simulink model "single_pendulum_R2018b"  (R2018b)
settings: Solver=ode1  StartTime=0.0  StopTime=60  FixedStep=0.01  MaxStep=0.1  RelTol=1e-3
settings Model: EnablePacing=on  Creator=mojo  LastModifiedBy=mojo
settings DataIOCC: ReturnWorkspaceOutputs=on

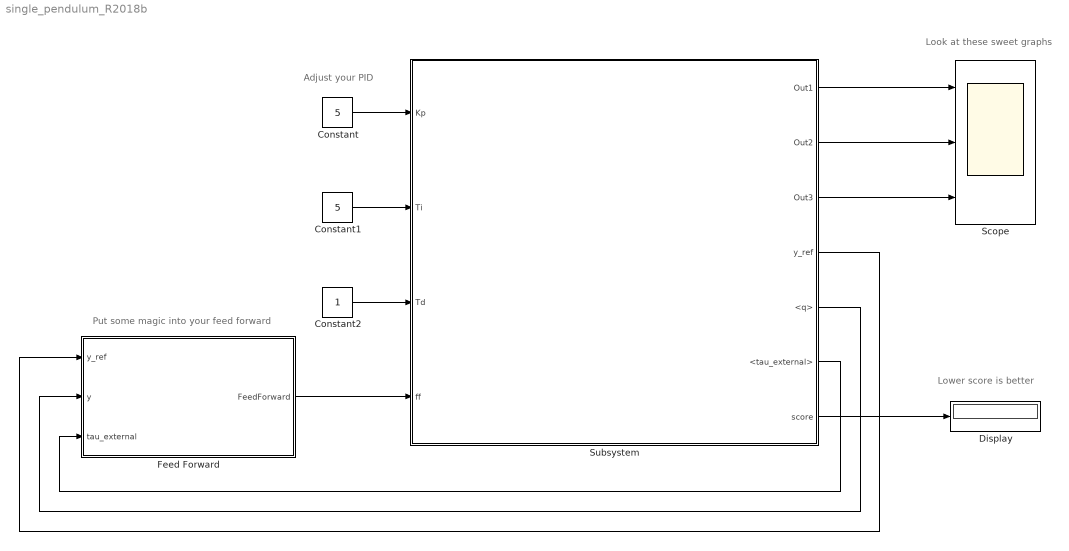
== system single_pendulum_R2018b ==
  note: Look at these sweet graphs
  note: Adjust your PID
  note: Put some magic into your feed forward
  note: Lower score is better
  Constant : Constant  Value=5
  Constant1 : Constant  Value=5
  Constant2 : Constant
  Display : Display
  Feed Forward : MATLAB Function  TreatAsAtomicUnit=on
  Scope : Scope  NumInputPorts=3
  Subsystem : Subsystem
  wires:
  Constant/1 -> Subsystem/1(Kp)
  Constant1/1 -> Subsystem/2(Ti)
  Constant2/1 -> Subsystem/3(Td)
  Feed Forward/1(FeedForward) -> Subsystem/4(ff)
  Subsystem/1(Out1) -> Scope/1
  Subsystem/2(Out2) -> Scope/2
  Subsystem/3(Out3) -> Scope/3
  Subsystem/4(y_ref) -> Feed Forward/1(y_ref)
  Subsystem/5(<q>) -> Feed Forward/2(y)
  Subsystem/6(<tau_external>) -> Feed Forward/3(tau_external)
  Subsystem/7(score) -> Display/1

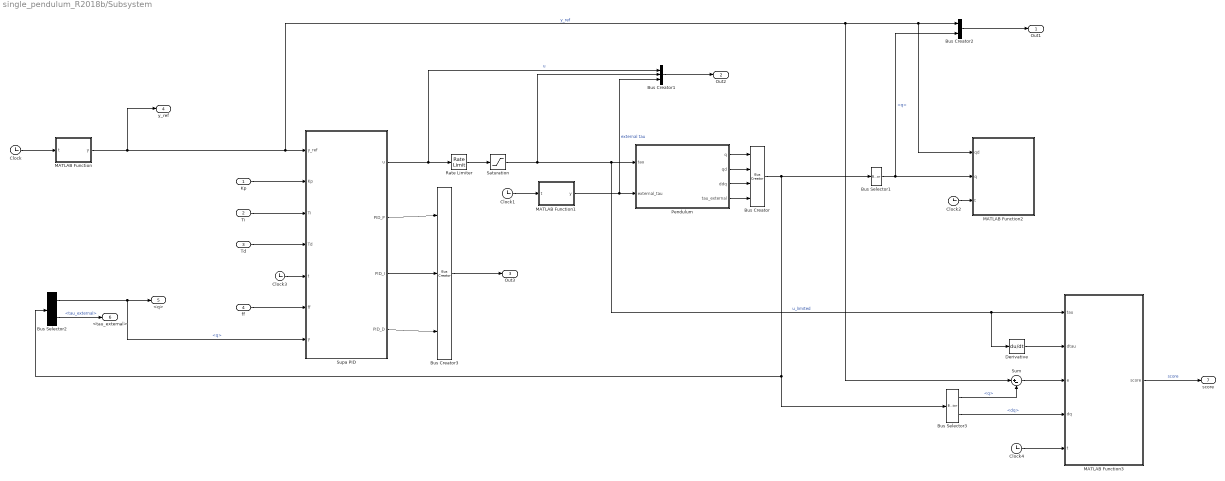
== system single_pendulum_R2018b/Subsystem ==
  Kp : Inport
  Ti : Inport  Port=2
  Td : Inport  Port=3
  ff : Inport  Port=4
  Bus Creator : BusCreator  Inputs=4
  Bus Creator1 : BusCreator  Inputs=3
  Bus Creator2 : BusCreator  Inputs=2
  Bus Creator3 : BusCreator  Inputs=3
  Bus Selector1 : BusSelector  OutputSignals=q
  Bus Selector2 : BusSelector  OutputSignals=q,tau_external
  Bus Selector3 : BusSelector  OutputSignals=q,dq
  Clock{,1..4} (5 alike) : Clock
  Derivative : Derivative
  MATLAB Function : MATLAB Function  TreatAsAtomicUnit=on
  MATLAB Function1 : MATLAB Function  TreatAsAtomicUnit=on
  MATLAB Function2 : MATLAB Function  TreatAsAtomicUnit=on
  MATLAB Function3 : MATLAB Function  TreatAsAtomicUnit=on
  Pendulum : Subsystem  mask{I=1, q_0=pi/2, Mass=1, Length=1, g=9.81, B=1}
      mask prompts: I "Inertia [kg*m]"; q_0 "Initial position [rad]"; Mass "Mass [kg]"; Length "Length [m]"; g "g [m/s^2]"; B "Friction [kg/s]"
  Rate Limiter : RateLimiter  RisingSlewLimit=20  FallingSlewLimit=-20  SampleTimeMode=inherited
  Saturation : Saturate  UpperLimit=30  LowerLimit=-30
  Sum : Sum  Inputs=|+-
  Supa PID : MATLAB Function  TreatAsAtomicUnit=on
  Out1 : Outport
  Out2 : Outport  Port=2
  Out3 : Outport  Port=3
  y_ref : Outport  Port=4
  <q> : Outport  Port=5
  <tau_external> : Outport  Port=6
  score : Outport  Port=7
  wires:
  Clock1/1 -> MATLAB Function1/1(t)
  Saturation/1 -> Bus Creator1/2, Derivative/1, MATLAB Function3/1(tau), Pendulum/1(tau)  "u_limited"
  MATLAB Function3/1(score) -> score/1  "score"
  Bus Creator/1 -> Bus Selector2/1, Bus Selector3/1, Bus Selector1/1
  Rate Limiter/1 -> Saturation/1
  MATLAB Function1/1(y) -> Bus Creator1/3, Pendulum/2(external_tau)  "external tau"
  Bus Selector1/1 -> MATLAB Function2/2(q), Bus Creator2/2  "<q>"
  Clock3/1 -> Supa PID/5(t)
  Bus Selector2/1 -> Supa PID/7(y), <q>/1  "<q>"
  ff/1 -> Supa PID/6(ff)
  MATLAB Function/1(y) -> y_ref/1, Sum/1, MATLAB Function2/1(qd), Bus Creator2/1, Supa PID/1(y_ref)  "y_ref"
  Supa PID/1(u) -> Rate Limiter/1, Bus Creator1/1  "u"
  Clock4/1 -> MATLAB Function3/5(t)
  Derivative/1 -> MATLAB Function3/2(dtau)
  Clock2/1 -> MATLAB Function2/3(t)
  Bus Selector3/1 -> Sum/2  "<q>"
  Bus Creator1/1 -> Out2/1
  Bus Selector2/2 -> <tau_external>/1  "<tau_external>"
  Sum/1 -> MATLAB Function3/3(e)
  Pendulum/1(q) -> Bus Creator/1
  Supa PID/2(PID_P) -> Bus Creator3/1
  Bus Selector3/2 -> MATLAB Function3/4(dq)  "<dq>"
  Supa PID/4(PID_D) -> Bus Creator3/3
  Pendulum/4("tau_external ") -> Bus Creator/4
  Supa PID/3(PID_I) -> Bus Creator3/2
  Clock/1 -> MATLAB Function/1(t)
  Pendulum/3(ddq) -> Bus Creator/3
  Pendulum/2(qd) -> Bus Creator/2
  Bus Creator2/1 -> Out1/1
  Ti/1 -> Supa PID/3(Ti)
  Kp/1 -> Supa PID/2(Kp)
  Bus Creator3/1 -> Out3/1
  Td/1 -> Supa PID/4(Td)

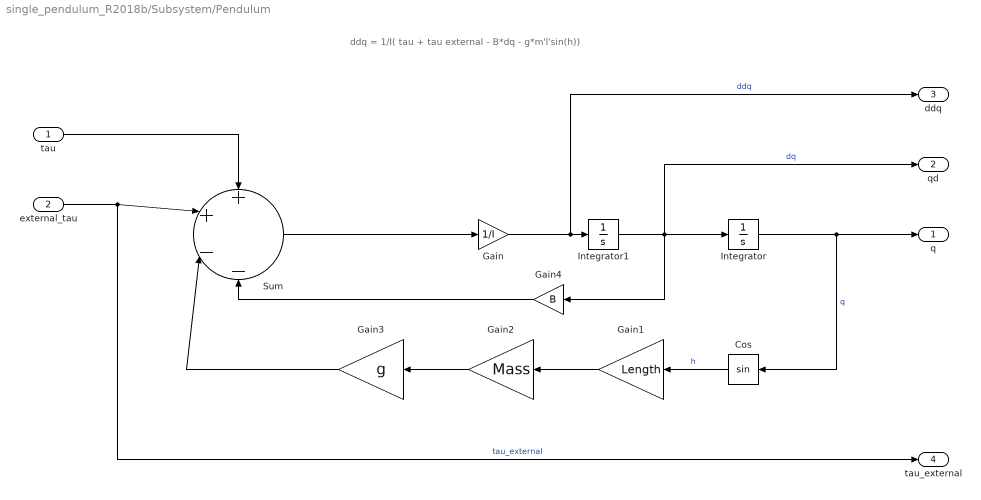
== system single_pendulum_R2018b/Subsystem/Pendulum ==
  note: ddq = 1/I( tau + tau external - B*dq - g*m'l'sin(h))
  tau : Inport
  external_tau : Inport  Port=2
  Cos : Trigonometry
  Gain : Gain  Gain=1/I
  Gain1 : Gain  Gain=Length
  Gain2 : Gain  Gain=Mass
  Gain3 : Gain  Gain=g
  Gain4 : Gain  Gain=B
  Integrator : Integrator  InitialCondition=q_0
  Integrator1 : Integrator
  Sum : Sum  Inputs=++--
  q : Outport
  qd : Outport  Port=2
  ddq : Outport  Port=3
  "tau_external " : Outport  Port=4
  wires:
  Integrator/1 -> Cos/1, q/1  "q"
  Integrator1/1 -> Gain4/1, qd/1, Integrator/1  "dq"
  Sum/1 -> Gain/1
  Gain/1 -> ddq/1, Integrator1/1  "ddq"
  tau/1 -> Sum/1
  external_tau/1 -> "tau_external "/1, Sum/2  "tau_external"
  Cos/1 -> Gain1/1  "h"
  Gain1/1 -> Gain2/1
  Gain2/1 -> Gain3/1
  Gain3/1 -> Sum/3
  Gain4/1 -> Sum/4

== matlab function single_pendulum_R2018b/Subsystem/Supa PID ==
  settings: updateMethod=DISCRETE
  data: y_ref input; Kp input; Ti input; Td input; t input; ff input; y input; u output; PID_P output; PID_I output; PID_D output
function [u, PID_P, PID_I, PID_D] = fcn(y_ref, Kp, Ti, Td, t, ff, y)
%% Supa dupa PID
% Without any clever stuff like anti-windup

%% Initialize
persistent y_prev e_prev t_prev I
if isempty(y_prev)
    y_prev = y;
    e_prev = 0;
    t_prev = t;
    I = 0;
    delta_t = 0.001;
else
    delta_t = t-t_prev;
end

%% Pre calc
e = y_ref - y;
dy = (y-y_prev)/delta_t;

%% I, D
if Ti>0
    I = I + delta_t*e/Ti;
else
    I = 0;
end

D = Td*(e-e_prev)/delta_t;

%% PID output
u = ff + Kp*(e + I + D);

%% Fun to look at.
PID_P = Kp*e;
PID_I = Kp*I;
PID_D = Kp*D;

%% Memory
y_prev = y;
e_prev = e;
t_prev = t;

== matlab function single_pendulum_R2018b/Subsystem/MATLAB Function ==
  data: t input; y output
function y = fcn(t)

if t < 5
    y = pi/2;
elseif t < 10
    y = 3*pi/4;
elseif t < 15
    y = 1*pi/4;
elseif t < 20
    y = 3*pi/4;
elseif t < 25
    y = 1*pi/4;
else
    y = pi/2;
end

== matlab function single_pendulum_R2018b/Subsystem/MATLAB Function1 ==
  data: t input; y output
function y = fcn(t)

if t < 30
    y = 0;
elseif t < 35
    y = 1;
elseif t < 40
    y = 0;
elseif t < 45
    y = -1;
elseif t < 50
    y = 0;
else
    y = 0;
end

== matlab function single_pendulum_R2018b/Feed Forward ==
  data: y_ref input; FeedForward output; y input; tau_external input
function FeedForward = fcn(y_ref, y, tau_external)


FeedForward = 0;

== matlab function single_pendulum_R2018b/Subsystem/MATLAB Function2 ==
  settings: updateMethod=DISCRETE
  data: qd input; q input; t input
function figure_that(qd, q, t)

frame_rate = 30; % [Hz]
persistent t_prev t_acc
if isempty(t_prev)
    t_prev = t;
    t_acc = 2/frame_rate;
end
t_acc = t_acc + (t-t_prev);
if t_acc > 1/frame_rate
    t_acc = 0;
    xd1 = sin(qd);
    yd1 = -cos(qd);
    
    x1 = sin(q);
    y1 = -cos(q);

    figure(2);
    clf;

    plot(0,0,'b*');
    hold on;
    plot([0,x1],[0,y1],'b');
    plot(x1,y1,'bo','LineWidth', 5);

    plot([0,xd1],[0,yd1],'g--','LineWidth', 2);

    axis([-2 2 -2 2]);
    grid on;
    title('Angles')
end

t_prev = t;

== matlab function single_pendulum_R2018b/Subsystem/MATLAB Function3 ==
  settings: updateMethod=DISCRETE
  data: tau input; score output; dtau input; e input; dq input; t input
function score  = fcn(tau, dtau, e, dq, t)

persistent t_prev score_prev
if isempty(t_prev)
    t_prev = 0;
    score_prev = 0;
    delta_t = 0.001;
else
    delta_t = t-t_prev;
end

score = score_prev + (...
    1*abs(e)/(2*pi/180) + 1*abs(dtau)/2 + 1*abs(tau)/15 ...
    )*delta_t;

%% Memory
t_prev = t;
score_prev = score;
